simulink model "nxtmouse"  (Simulink 6.4)
settings: Solver=ode4  StartTime=0.0  StopTime=inf  FixedStep=Ts  RelTol=1e-3
PreLoadFcn:
  | param;
values from neighbouring files (symbols this model uses):
  CAMERA_POS = [100 100]    [param.m]
  Cm = 9.00e-6    (= 9e-06)    [param.m]
  Cw = 9.00e-4    (= 0.0009)    [param.m]
  Dx = 1e-3    (= 0.001)    [param.m]
  Dzz = 1e-6    (= 1e-06)    [param.m]
  e = -0.2    [param.m]
  J = M*(W/2)^2    (= 0.004096)    [param.m]
  Jm = 0.5e-7    (= 5e-08)    [param.m]
  Jw = 20.0e-7    (= 2e-06)    [param.m]
  Kb = 0.022    [param.m]
  Kt = 0.022    [param.m]
  LENGTH = 20    [param.m]
  LENGTH2 = 16    [param.m]
  Lm = 1.4e-3    (= 0.0014)    [param.m]
  M = 0.64    [param.m]
  n = 24    [param.m]
  Rm = 1.0    (= 1)    [param.m]
  Rw = 0.056/2    (= 0.028)    [param.m]
  START_POS = [22 15]    [param.m]
  TRACK_MAP = double(imread('track.bmp'))    [param.m]
  Ts = 0.0001    [param.m]
  W = 0.16    [param.m]
  WALL_MAP = ~(TRACK_MAP - WALL)    [param.m]
  WIDTH = 16    [param.m]
  WIDTH1 = 12    [param.m]
undefined symbols (not defined in the file or in its folder): clearNXTSignalObjects, DiscIntNeverNeededParam
libraries: simulink x13, vrlib x1, ecrobot_nxt_lib x1
(part 3 of 3)

== system nxtmouse/Virtual_Track/Wall hit dection/Wall hit FR/If Action Subsystem1 ==
  Action Port : ActionPort  ActionType=else
  Constant : Constant  Value=1  OutDataType=sfix(16)  ConRadixGroup=Use specified scaling  OutScaling=2^0  SampleTime=inf  FramePeriod=inf
  Stop Simulation : Stop
  wires:
  Constant/1 -> Stop Simulation/1

== system nxtmouse/Virtual_Track/Wall hit dection/Wall hit RC/If Action Subsystem ==
  z : Inport
  x : Inport  Port=2
  Action Port : ActionPort  ActionType=then
  Constant1 : Constant  Value=1  OutDataType=sfix(16)  ConRadixGroup=Use specified scaling  OutScaling=2^0  SampleTime=inf  FramePeriod=inf
  Constant5 : Constant  Value=size(TRACK_MAP,1)  OutDataType=sfix(16)  ConRadixGroup=Use specified scaling  OutScaling=2^0  SampleTime=inf  FramePeriod=inf
  Direct Lookup Table (n-D) : simulink/Lookup Tables/Direct Lookup Table (n-D)  maskTabDims=2  explicitNumDims=1  outDims=Element  tabIsInput=off  mxTable=WALL_MAP(:,:,1)  clipFlag=Warning
  Saturation : Saturate  UpperLimit=200  LowerLimit=1
  Saturation1 : Saturate  UpperLimit=200  LowerLimit=1
  Sum1 : Sum  Inputs=-+|
  Sum2 : Sum  Inputs=|+-
  Sum4 : Sum  Inputs=+-|
  Out1 : Outport
  wires:
  Direct Lookup Table (n-D)/1 -> Out1/1
  z/1 -> Sum2/1
  Constant1/1 -> Sum2/2, Sum1/1
  x/1 -> Sum1/2
  Sum2/1 -> Saturation/1
  Sum1/1 -> Saturation1/1
  Saturation1/1 -> Direct Lookup Table (n-D)/2
  Saturation/1 -> Sum4/2
  Constant5/1 -> Sum4/1
  Sum4/1 -> Direct Lookup Table (n-D)/1

== system nxtmouse/Virtual_Track/Wall hit dection/Wall hit RC/If Action Subsystem1 ==
  Action Port : ActionPort  ActionType=else
  Constant : Constant  Value=1  OutDataType=sfix(16)  ConRadixGroup=Use specified scaling  OutScaling=2^0  SampleTime=inf  FramePeriod=inf
  Stop Simulation : Stop
  wires:
  Constant/1 -> Stop Simulation/1

== system nxtmouse/Virtual_Track/Wall hit dection/Wall hit RL/If Action Subsystem ==
  z : Inport
  x : Inport  Port=2
  Action Port : ActionPort  ActionType=then
  Constant1 : Constant  Value=1  OutDataType=sfix(16)  ConRadixGroup=Use specified scaling  OutScaling=2^0  SampleTime=inf  FramePeriod=inf
  Constant5 : Constant  Value=size(TRACK_MAP,1)  OutDataType=sfix(16)  ConRadixGroup=Use specified scaling  OutScaling=2^0  SampleTime=inf  FramePeriod=inf
  Direct Lookup Table (n-D) : simulink/Lookup Tables/Direct Lookup Table (n-D)  maskTabDims=2  explicitNumDims=1  outDims=Element  tabIsInput=off  mxTable=WALL_MAP(:,:,1)  clipFlag=Warning
  Saturation : Saturate  UpperLimit=200  LowerLimit=1
  Saturation1 : Saturate  UpperLimit=200  LowerLimit=1
  Sum1 : Sum  Inputs=-+|
  Sum2 : Sum  Inputs=|+-
  Sum4 : Sum  Inputs=+-|
  Out1 : Outport
  wires:
  Direct Lookup Table (n-D)/1 -> Out1/1
  z/1 -> Sum2/1
  Constant1/1 -> Sum2/2, Sum1/1
  x/1 -> Sum1/2
  Sum2/1 -> Saturation/1
  Sum1/1 -> Saturation1/1
  Saturation1/1 -> Direct Lookup Table (n-D)/2
  Saturation/1 -> Sum4/2
  Constant5/1 -> Sum4/1
  Sum4/1 -> Direct Lookup Table (n-D)/1

== system nxtmouse/Virtual_Track/Wall hit dection/Wall hit RL/If Action Subsystem1 ==
  Action Port : ActionPort  ActionType=else
  Constant : Constant  Value=1  OutDataType=sfix(16)  ConRadixGroup=Use specified scaling  OutScaling=2^0  SampleTime=inf  FramePeriod=inf
  Stop Simulation : Stop
  wires:
  Constant/1 -> Stop Simulation/1

== system nxtmouse/Virtual_Track/Wall hit dection/Wall hit RR/If Action Subsystem ==
  z : Inport
  x : Inport  Port=2
  Action Port : ActionPort  ActionType=then
  Constant1 : Constant  Value=1  OutDataType=sfix(16)  ConRadixGroup=Use specified scaling  OutScaling=2^0  SampleTime=inf  FramePeriod=inf
  Constant5 : Constant  Value=size(TRACK_MAP,1)  OutDataType=sfix(16)  ConRadixGroup=Use specified scaling  OutScaling=2^0  SampleTime=inf  FramePeriod=inf
  Direct Lookup Table (n-D) : simulink/Lookup Tables/Direct Lookup Table (n-D)  maskTabDims=2  explicitNumDims=1  outDims=Element  tabIsInput=off  mxTable=WALL_MAP(:,:,1)  clipFlag=Warning
  Saturation : Saturate  UpperLimit=200  LowerLimit=1
  Saturation1 : Saturate  UpperLimit=200  LowerLimit=1
  Sum1 : Sum  Inputs=-+|
  Sum2 : Sum  Inputs=|+-
  Sum4 : Sum  Inputs=+-|
  Out1 : Outport
  wires:
  Sum4/1 -> Direct Lookup Table (n-D)/1
  Constant5/1 -> Sum4/1
  Saturation/1 -> Sum4/2
  Saturation1/1 -> Direct Lookup Table (n-D)/2
  Sum1/1 -> Saturation1/1
  Sum2/1 -> Saturation/1
  x/1 -> Sum1/2
  Constant1/1 -> Sum1/1, Sum2/2
  z/1 -> Sum2/1
  Direct Lookup Table (n-D)/1 -> Out1/1

== system nxtmouse/Virtual_Track/Wall hit dection/Wall hit RR/If Action Subsystem1 ==
  Action Port : ActionPort  ActionType=else
  Constant : Constant  Value=1  OutDataType=sfix(16)  ConRadixGroup=Use specified scaling  OutScaling=2^0  SampleTime=inf  FramePeriod=inf
  Stop Simulation : Stop
  wires:
  Constant/1 -> Stop Simulation/1

== system nxtmouse/Virtual_Track/Light Sensor L/Subsystem/Sensing FR/If Action Subsystem ==
  z : Inport
  x : Inport  Port=2
  Action Port : ActionPort  ActionType=then
  Constant1 : Constant  Value=1  OutDataType=sfix(16)  ConRadixGroup=Use specified scaling  OutScaling=2^0  SampleTime=inf  FramePeriod=inf
  Constant5 : Constant  Value=size(TRACK_MAP,1)  OutDataType=sfix(16)  ConRadixGroup=Use specified scaling  OutScaling=2^0  SampleTime=inf  FramePeriod=inf
  Direct Lookup Table (n-D) : simulink/Lookup Tables/Direct Lookup Table (n-D)  maskTabDims=2  explicitNumDims=1  outDims=Element  tabIsInput=off  mxTable=WALL_MAP(:,:,1)  clipFlag=Warning
  Saturation : Saturate  UpperLimit=200  LowerLimit=1
  Saturation1 : Saturate  UpperLimit=200  LowerLimit=1
  Sum1 : Sum  Inputs=-+|
  Sum2 : Sum  Inputs=|+-
  Sum4 : Sum  Inputs=+-|
  Out1 : Outport  InitialOutput=0
  wires:
  Sum4/1 -> Direct Lookup Table (n-D)/1
  Constant5/1 -> Sum4/1
  Saturation/1 -> Sum4/2
  Saturation1/1 -> Direct Lookup Table (n-D)/2
  Sum1/1 -> Saturation1/1
  Sum2/1 -> Saturation/1
  x/1 -> Sum1/2
  Constant1/1 -> Sum1/1, Sum2/2
  z/1 -> Sum2/1
  Direct Lookup Table (n-D)/1 -> Out1/1

== system nxtmouse/Virtual_Track/Light Sensor L/Subsystem/Sensing FR/If Action Subsystem1 ==
  Action Port : ActionPort  ActionType=else
  Constant : Constant  Value=0  OutDataTypeMode=boolean  OutDataType=sfix(16)  ConRadixGroup=Use specified scaling  OutScaling=2^0  SampleTime=inf  FramePeriod=inf
  Out1 : Outport  InitialOutput=0
  wires:
  Constant/1 -> Out1/1

== system nxtmouse/Virtual_Track/Light Sensor R/Subsystem/Sensing FR/If Action Subsystem ==
  z : Inport
  x : Inport  Port=2
  Action Port : ActionPort  ActionType=then
  Constant1 : Constant  Value=1  OutDataType=sfix(16)  ConRadixGroup=Use specified scaling  OutScaling=2^0  SampleTime=inf  FramePeriod=inf
  Constant5 : Constant  Value=size(TRACK_MAP,1)  OutDataType=sfix(16)  ConRadixGroup=Use specified scaling  OutScaling=2^0  SampleTime=inf  FramePeriod=inf
  Direct Lookup Table (n-D) : simulink/Lookup Tables/Direct Lookup Table (n-D)  maskTabDims=2  explicitNumDims=1  outDims=Element  tabIsInput=off  mxTable=WALL_MAP(:,:,1)  clipFlag=Warning
  Saturation : Saturate  UpperLimit=200  LowerLimit=1
  Saturation1 : Saturate  UpperLimit=200  LowerLimit=1
  Sum1 : Sum  Inputs=-+|
  Sum2 : Sum  Inputs=|+-
  Sum4 : Sum  Inputs=+-|
  Out1 : Outport  InitialOutput=0
  wires:
  Sum4/1 -> Direct Lookup Table (n-D)/1
  Constant5/1 -> Sum4/1
  Saturation/1 -> Sum4/2
  Saturation1/1 -> Direct Lookup Table (n-D)/2
  Sum1/1 -> Saturation1/1
  Sum2/1 -> Saturation/1
  x/1 -> Sum1/2
  Constant1/1 -> Sum1/1, Sum2/2
  z/1 -> Sum2/1
  Direct Lookup Table (n-D)/1 -> Out1/1

== system nxtmouse/Virtual_Track/Light Sensor R/Subsystem/Sensing FR/If Action Subsystem1 ==
  Action Port : ActionPort  ActionType=else
  Constant : Constant  Value=0  OutDataTypeMode=boolean  OutDataType=sfix(16)  ConRadixGroup=Use specified scaling  OutScaling=2^0  SampleTime=inf  FramePeriod=inf
  Out1 : Outport  InitialOutput=0
  wires:
  Constant/1 -> Out1/1

== system nxtmouse/Virtual_Track/Ultrasonic Sensor/Subsystem/Sensing FC/If Action Subsystem ==
  z : Inport
  x : Inport  Port=2
  Action Port : ActionPort  ActionType=then
  Constant1 : Constant  Value=1  OutDataType=sfix(16)  ConRadixGroup=Use specified scaling  OutScaling=2^0  SampleTime=inf  FramePeriod=inf
  Constant5 : Constant  Value=size(TRACK_MAP,1)  OutDataType=sfix(16)  ConRadixGroup=Use specified scaling  OutScaling=2^0  SampleTime=inf  FramePeriod=inf
  Direct Lookup Table (n-D) : simulink/Lookup Tables/Direct Lookup Table (n-D)  maskTabDims=2  explicitNumDims=1  outDims=Element  tabIsInput=off  mxTable=WALL_MAP(:,:,1)  clipFlag=Warning
  Saturation : Saturate  UpperLimit=200  LowerLimit=1
  Saturation1 : Saturate  UpperLimit=200  LowerLimit=1
  Sum1 : Sum  Inputs=-+|
  Sum2 : Sum  Inputs=|+-
  Sum4 : Sum  Inputs=+-|
  Out1 : Outport  InitialOutput=0
  wires:
  Sum4/1 -> Direct Lookup Table (n-D)/1
  Constant5/1 -> Sum4/1
  Saturation/1 -> Sum4/2
  Saturation1/1 -> Direct Lookup Table (n-D)/2
  Sum1/1 -> Saturation1/1
  Sum2/1 -> Saturation/1
  x/1 -> Sum1/2
  Constant1/1 -> Sum1/1, Sum2/2
  z/1 -> Sum2/1
  Direct Lookup Table (n-D)/1 -> Out1/1

== system nxtmouse/Virtual_Track/Ultrasonic Sensor/Subsystem/Sensing FC/If Action Subsystem1 ==
  Action Port : ActionPort  ActionType=else
  Constant : Constant  Value=0  OutDataTypeMode=boolean  OutDataType=sfix(16)  ConRadixGroup=Use specified scaling  OutScaling=2^0  SampleTime=inf  FramePeriod=inf
  Out1 : Outport  InitialOutput=0
  wires:
  Constant/1 -> Out1/1

== system nxtmouse/Virtual_Track/Ultrasonic Sensor/Subsystem/Sensing FL/If Action Subsystem ==
  z : Inport
  x : Inport  Port=2
  Action Port : ActionPort  ActionType=then
  Constant1 : Constant  Value=1  OutDataType=sfix(16)  ConRadixGroup=Use specified scaling  OutScaling=2^0  SampleTime=inf  FramePeriod=inf
  Constant5 : Constant  Value=size(TRACK_MAP,1)  OutDataType=sfix(16)  ConRadixGroup=Use specified scaling  OutScaling=2^0  SampleTime=inf  FramePeriod=inf
  Direct Lookup Table (n-D) : simulink/Lookup Tables/Direct Lookup Table (n-D)  maskTabDims=2  explicitNumDims=1  outDims=Element  tabIsInput=off  mxTable=WALL_MAP(:,:,1)  clipFlag=Warning
  Saturation : Saturate  UpperLimit=200  LowerLimit=1
  Saturation1 : Saturate  UpperLimit=200  LowerLimit=1
  Sum1 : Sum  Inputs=-+|
  Sum2 : Sum  Inputs=|+-
  Sum4 : Sum  Inputs=+-|
  Out1 : Outport  InitialOutput=0
  wires:
  Direct Lookup Table (n-D)/1 -> Out1/1
  z/1 -> Sum2/1
  Constant1/1 -> Sum2/2, Sum1/1
  x/1 -> Sum1/2
  Sum2/1 -> Saturation/1
  Sum1/1 -> Saturation1/1
  Saturation1/1 -> Direct Lookup Table (n-D)/2
  Saturation/1 -> Sum4/2
  Constant5/1 -> Sum4/1
  Sum4/1 -> Direct Lookup Table (n-D)/1

== system nxtmouse/Virtual_Track/Ultrasonic Sensor/Subsystem/Sensing FL/If Action Subsystem1 ==
  Action Port : ActionPort  ActionType=else
  Constant : Constant  Value=0  OutDataTypeMode=boolean  OutDataType=sfix(16)  ConRadixGroup=Use specified scaling  OutScaling=2^0  SampleTime=inf  FramePeriod=inf
  Out1 : Outport  InitialOutput=0
  wires:
  Constant/1 -> Out1/1

== system nxtmouse/Virtual_Track/Ultrasonic Sensor/Subsystem/Sensing FR/If Action Subsystem ==
  z : Inport
  x : Inport  Port=2
  Action Port : ActionPort  ActionType=then
  Constant1 : Constant  Value=1  OutDataType=sfix(16)  ConRadixGroup=Use specified scaling  OutScaling=2^0  SampleTime=inf  FramePeriod=inf
  Constant5 : Constant  Value=size(TRACK_MAP,1)  OutDataType=sfix(16)  ConRadixGroup=Use specified scaling  OutScaling=2^0  SampleTime=inf  FramePeriod=inf
  Direct Lookup Table (n-D) : simulink/Lookup Tables/Direct Lookup Table (n-D)  maskTabDims=2  explicitNumDims=1  outDims=Element  tabIsInput=off  mxTable=WALL_MAP(:,:,1)  clipFlag=Warning
  Saturation : Saturate  UpperLimit=200  LowerLimit=1
  Saturation1 : Saturate  UpperLimit=200  LowerLimit=1
  Sum1 : Sum  Inputs=-+|
  Sum2 : Sum  Inputs=|+-
  Sum4 : Sum  Inputs=+-|
  Out1 : Outport  InitialOutput=0
  wires:
  Direct Lookup Table (n-D)/1 -> Out1/1
  z/1 -> Sum2/1
  Constant1/1 -> Sum2/2, Sum1/1
  x/1 -> Sum1/2
  Sum2/1 -> Saturation/1
  Sum1/1 -> Saturation1/1
  Saturation1/1 -> Direct Lookup Table (n-D)/2
  Saturation/1 -> Sum4/2
  Constant5/1 -> Sum4/1
  Sum4/1 -> Direct Lookup Table (n-D)/1

== system nxtmouse/Virtual_Track/Ultrasonic Sensor/Subsystem/Sensing FR/If Action Subsystem1 ==
  Action Port : ActionPort  ActionType=else
  Constant : Constant  Value=0  OutDataTypeMode=boolean  OutDataType=sfix(16)  ConRadixGroup=Use specified scaling  OutScaling=2^0  SampleTime=inf  FramePeriod=inf
  Out1 : Outport  InitialOutput=0
  wires:
  Constant/1 -> Out1/1

== system nxtmouse/Virtual_Track/Virtual Reality/calc rear tyre assy rot/calc rear tyre rev/Triggered Subsystem ==
  Trigger : TriggerPort  TriggerType=either
  Constant : Constant  Value=-1  OutDataType=sfix(16)  ConRadixGroup=Use specified scaling  OutScaling=2^0  SampleTime=inf  FramePeriod=inf
  Product : Product  RndMeth=Zero
  Unit Delay : UnitDelay  Orientation=left  X0=-1  SampleTime=-1
  Out1 : Outport
  wires:
  Constant/1 -> Product/1
  Product/1 -> Out1/1, Unit Delay/1
  Unit Delay/1 -> Product/2

== stateflow chart Virtual_Track/Ultrasonic Sensor/Iterator ==
  (junction 4) -> (junction 10) [order 2] : {
      |  distance = range+noise;
      | }
  (junction 3) -> (junction 4) : {
      |  SearchObstacle;
      | }
  (junction 4) -> (junction 5) [order 1] : [obstacle == 0]
  (junction 15) -> (junction 6) : {
      |  range = range + 1;
      | }
  (junction 6) -> (junction 3)
  (junction 16) -> (junction 13)
  (junction 10) -> (junction 8) [order 1] : [distance > 255+offset]
  (junction 8) -> (junction 13) : {
      |  distance = ...
      |  255 + offset;
      | }
  (junction 9) -> (junction 7) [order 2]
  (junction 11) -> (junction 7)
  (junction 13) -> (junction 11)
  (junction 12) -> (junction 11) : {
      |  distance = offset;
      | }
  (junction 9) -> (junction 12) [order 1] : [distance < offset]
  (junction 10) -> (junction 9) [order 2]
  (junction 5) -> (junction 14)
  (junction 14) -> (junction 15) [order 1] : [range < 256+offset]
  (junction 14) -> (junction 16) [order 2] : {
      |  distance = ...
      |   255+offset;
      | }
  (default) -> (junction 18) : {
      |  range = offset+1;
      |  distance = 0;
      | }
  (junction 20) -> (junction 17)
  (junction 18) -> (junction 19) [order 1] : [(rotation > 3.14/12 && rotation < 3.14*5/12) && noise > 0]
  (junction 19) -> (junction 20) : {
      | range_cnt = -1;
      | }
  (junction 18) -> (junction 17) [order 2] : {
      |  range_cnt = 0;
      | }
  (junction 17) -> (junction 3)
  (junction 7) -> (junction 21) : {
      | range_cnt = range_cnt + 1;
      | }
  (junction 21) -> (junction 22) [order 1] : [range_cnt < 1 && (distance >= 0 && distance <=(255+offset))]
  (junction 22) -> (junction 15) : {
      |  range = range + 2;
      | }
  (junction 21) -> (junction 23) [order 2] : {
      | distance = distance - offset;
      | }
  data: range output double; obstacle input inherited; offset input double; distance output double =255; noise input double; rotation input double; range_cnt local double
  events: SearchObstacle output FUNCTION_CALL_EVENT

== stateflow chart Virtual_Track/Light Sensor R/Iterator ==
  (junction 62) -> (junction 68) [order 2] : {
      |  distance = range+noise;
      | }
  (junction 61) -> (junction 62) : {
      |  SearchObstacle;
      | }
  (junction 62) -> (junction 63) [order 1] : [obstacle == 0]
  (junction 73) -> (junction 64) : {
      |  range = range + 1;
      | }
  (junction 64) -> (junction 61)
  (junction 74) -> (junction 71)
  (junction 68) -> (junction 66) [order 1] : [distance > 50]
  (junction 66) -> (junction 71) : {
      |  distance = 50;
      | }
  (junction 67) -> (junction 65) [order 2]
  (junction 69) -> (junction 65)
  (junction 71) -> (junction 69)
  (junction 70) -> (junction 69) : {
      |  distance = 0;
      | }
  (junction 67) -> (junction 70) [order 1] : [distance < 0]
  (junction 68) -> (junction 67) [order 2]
  (junction 63) -> (junction 72)
  (junction 72) -> (junction 73) [order 1] : [range < 51]
  (junction 72) -> (junction 74) [order 2] : {
      |  distance = 50;
      | }
  (default) -> (junction 76) : {
      |  range = 1;
      |  distance = 0;
      | }
  (junction 78) -> (junction 75)
  (junction 76) -> (junction 77) [order 1] : [(rotation > 3.14/12 && rotation < 3.14*5/12) && noise > 0]
  (junction 77) -> (junction 78) : {
      | range_cnt = -1;
      | }
  (junction 76) -> (junction 75) [order 2] : {
      |  range_cnt = 0;
      | }
  (junction 75) -> (junction 61)
  (junction 65) -> (junction 79) : {
      | range_cnt = range_cnt + 1;
      | }
  (junction 79) -> (junction 80) [order 1] : [range_cnt < 1 && (distance >= 0 && distance <=50)]
  (junction 80) -> (junction 73) : {
      |  range = range + 2;
      | }
  (junction 79) -> (junction 81) [order 2]
  data: range output double; obstacle input inherited; distance output double; noise input double; rotation input double; range_cnt local double
  events: SearchObstacle output FUNCTION_CALL_EVENT

== stateflow chart Virtual_Track/Light Sensor L/Iterator ==
  (junction 119) -> (junction 125) [order 2] : {
      |  distance = range+noise;
      | }
  (junction 118) -> (junction 119) : {
      |  SearchObstacle;
      | }
  (junction 119) -> (junction 120) [order 1] : [obstacle == 0]
  (junction 130) -> (junction 121) : {
      |  range = range + 1;
      | }
  (junction 121) -> (junction 118)
  (junction 131) -> (junction 128)
  (junction 125) -> (junction 123) [order 1] : [distance > 50]
  (junction 123) -> (junction 128) : {
      |  distance = 50;
      | }
  (junction 124) -> (junction 122) [order 2]
  (junction 126) -> (junction 122)
  (junction 128) -> (junction 126)
  (junction 127) -> (junction 126) : {
      |  distance = 0;
      | }
  (junction 124) -> (junction 127) [order 1] : [distance < 0]
  (junction 125) -> (junction 124) [order 2]
  (junction 120) -> (junction 129)
  (junction 129) -> (junction 130) [order 1] : [range < 51]
  (junction 129) -> (junction 131) [order 2] : {
      |  distance = 50;
      | }
  (default) -> (junction 133) : {
      |  range = 1;
      |  distance = 0;
      | }
  (junction 135) -> (junction 132)
  (junction 133) -> (junction 134) [order 1] : [(rotation > 3.14/12 && rotation < 3.14*5/12) && noise > 0]
  (junction 134) -> (junction 135) : {
      | range_cnt = -1;
      | }
  (junction 133) -> (junction 132) [order 2] : {
      |  range_cnt = 0;
      | }
  (junction 132) -> (junction 118)
  (junction 122) -> (junction 136) : {
      | range_cnt = range_cnt + 1;
      | }
  (junction 136) -> (junction 137) [order 1] : [range_cnt < 1 && (distance >= 0 && distance <=50)]
  (junction 137) -> (junction 130) : {
      |  range = range + 2;
      | }
  (junction 136) -> (junction 138) [order 2]
  data: range output double; obstacle input inherited; distance output double; noise input double; rotation input double; range_cnt local double
  events: SearchObstacle output FUNCTION_CALL_EVENT
